simulink model "Slink__Analog_Buck_Control"  (R2023b)
settings: Solver=VariableStepAuto  StartTime=0.0  StopTime=1  RelTol=1e-6
values from neighbouring files (symbols this model uses):
  C = 22e-6    (= 2.2e-05)    [Final_Project.m]
  C2_c = 1e-6    (= 1e-06)    [Final_Project.m]
  fs = 12e3    (= 12000)    [Final_Project.m]
  L = 1e-3    (= 0.001)    [Final_Project.m]
  R = 22    [Final_Project.m]
  R1 = 20e3    (= 20000)    [Final_Project.m]
  R1_c = 10e3    (= 10000)    [Final_Project.m]
  R2 = Hs*R1    (= 2000)    [Final_Project.m]
  R3_c = 10e3    (= 10000)    [Final_Project.m]
  R4_c = 3.9e3    (= 3900)    [Final_Project.m]
  Vd = 36*sqrt(2)    [Final_Project.m]
libraries: spsSeriesRLCBranchLib x23, spsGroundLib x11, spsVoltageMeasurementLib x9, spsControlledVoltageSourceLib x6, simulink x4, spsCurrentMeasurementLib x1, spsDiodeLib x1, spsIdealSwitchLib x1, spsMeanLib x1, eePwmGenerator x1, spspowerguiLib x1
settings Model: Creator=Lucas  LastModifiedBy=Lucas

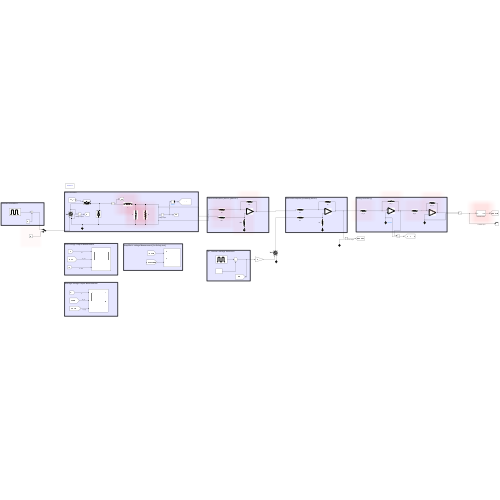
[thumbnail: Simulink's stored preview of the top-level diagram]
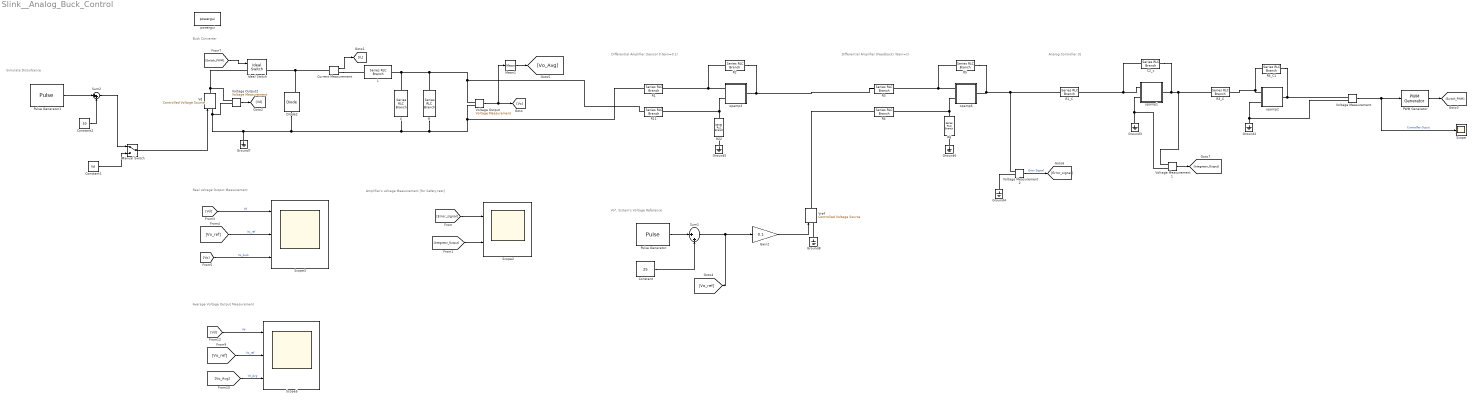
== system Slink__Analog_Buck_Control ==
  note: Amplifier's voltage Measurement [for Safety test]
  note: Vo*, Sistem's Voltage Reference
  note: Simulate Disturbance
  note: Differential Amplifier [Feedback] (Gain=1)
  note: Analog Controller [I]
  note: Differential Amplifier [Sensor ](Gain=0.1)
  note: Buck Converter
  note: Average Voltage Output Measurement
  note: Real voltage Output Measurement
  C : spsSeriesRLCBranchLib/Series RLC Branch  LConnTagsString=__new0  RConnTagsString=__new0  BranchType=C  Resistance=1  Inductance=L  SetiL0=off  InitialCurrent=0  Capacitance=C  Setx0=off  InitialVoltage=0  Measurements=None
  C2_c : spsSeriesRLCBranchLib/Series RLC Branch  LConnTagsString=__new0  RConnTagsString=__new0  BranchType=C  Resistance=R2  Inductance=1e-3  SetiL0=off  InitialCurrent=0  Capacitance=C2_c  Setx0=off  InitialVoltage=0  Measurements=None
  Constant : Constant  Value=25
  Constant1 : Constant  Value=Vd
  Constant2 : Constant  Value=50
  Current Measurement : spsCurrentMeasurementLib/Current Measurement  PhasorSimulation=off  OutputType=Complex  PSBequivalent=0
  Diode2 : spsDiodeLib/Diode  Ron=0.00001  Lon=0  Vf=0  IC=0  UseSnubber=0  Rs=inf  Cs=inf  Measurements=on
  Gain2 : Gain  Gain=0.1
  Ground{2..8} (7 alike) : spsGroundLib/Ground  LConnTagsString=a
  Ideal Switch : spsIdealSwitchLib/Ideal Switch  Ron=0.001  Lon=0  IC=0  Rs=1e5  Cs=inf  Measurements=on
  L : spsSeriesRLCBranchLib/Series RLC Branch  LConnTagsString=__new0  RConnTagsString=__new0  BranchType=L  Resistance=1  Inductance=L  SetiL0=off  InitialCurrent=0  Capacitance=1e-6  Setx0=off  InitialVoltage=0  Measurements=None
  Manual Switch : ManualSwitch
  Mean1 : spsMeanLib/Mean  Freq=60  Vinit=0  Ts=0
  PWM Generator : eePwmGenerator/PWM Generator  CarrCount=Up  Tper=1/fs  Tdelay=0  Ts=0
  Pulse Generator : DiscretePulseGenerator  PulseType=Time based  Amplitude=20  Period=0.5  PulseWidth=50  PhaseDelay=0.2
  Pulse Generator1 : DiscretePulseGenerator  PulseType=Time based  Amplitude=20  Period=0.5  PulseWidth=50  PhaseDelay=0.1
  R : spsSeriesRLCBranchLib/Series RLC Branch  LConnTagsString=__new0  RConnTagsString=__new0  BranchType=R  Resistance=R  Inductance=L  SetiL0=off  InitialCurrent=0  Capacitance=1e-6  Setx0=off  InitialVoltage=0  Measurements=None
  R1 : spsSeriesRLCBranchLib/Series RLC Branch  LConnTagsString=__new0  RConnTagsString=__new0  BranchType=R  Resistance=R1  Inductance=1e-3  SetiL0=off  InitialCurrent=0  Capacitance=1e-6  Setx0=off  InitialVoltage=0  Measurements=None
  R11 : spsSeriesRLCBranchLib/Series RLC Branch  LConnTagsString=__new0  RConnTagsString=__new0  BranchType=R  Resistance=R1  Inductance=1e-3  SetiL0=off  InitialCurrent=0  Capacitance=1e-6  Setx0=off  InitialVoltage=0  Measurements=None
  R1_C : spsSeriesRLCBranchLib/Series RLC Branch  LConnTagsString=__new0  RConnTagsString=__new0  BranchType=R  Resistance=R1_c  Inductance=1e-3  SetiL0=off  InitialCurrent=0  Capacitance=1e-6  Setx0=off  InitialVoltage=0  Measurements=None
  R2 : spsSeriesRLCBranchLib/Series RLC Branch  LConnTagsString=__new0  RConnTagsString=__new0  BranchType=R  Resistance=R2  Inductance=1e-3  SetiL0=off  InitialCurrent=0  Capacitance=1e-6  Setx0=off  InitialVoltage=0  Measurements=None
  R22 : spsSeriesRLCBranchLib/Series RLC Branch  LConnTagsString=__new0  RConnTagsString=__new0  BranchType=R  Resistance=R2  Inductance=1e-3  SetiL0=off  InitialCurrent=0  Capacitance=1e-6  Setx0=off  InitialVoltage=0  Measurements=None
  R{3..6} (4 alike) : spsSeriesRLCBranchLib/Series RLC Branch  LConnTagsString=__new0  RConnTagsString=__new0  BranchType=R  Resistance=2e3  Inductance=1e-3  SetiL0=off  InitialCurrent=0  Capacitance=1e-6  Setx0=off  InitialVoltage=0  Measurements=None
  R3_C : spsSeriesRLCBranchLib/Series RLC Branch  LConnTagsString=__new0  RConnTagsString=__new0  BranchType=R  Resistance=R3_c  Inductance=1e-3  SetiL0=off  InitialCurrent=0  Capacitance=1e-6  Setx0=off  InitialVoltage=0  Measurements=None
  R4_C1 : spsSeriesRLCBranchLib/Series RLC Branch  LConnTagsString=__new0  RConnTagsString=__new0  BranchType=R  Resistance=R4_c  Inductance=1e-3  SetiL0=off  InitialCurrent=0  Capacitance=1e-6  Setx0=off  InitialVoltage=0  Measurements=None
  Scope : Scope
  Scope2 : Scope  NumInputPorts=2
  Scope3 : Scope  NumInputPorts=3
  Scope5 : Scope  NumInputPorts=3
  Sum1 : Sum  Inputs=|++
  Sum2 : Sum  Inputs=|++
  Vd : spsControlledVoltageSourceLib/Controlled Voltage Source  Initialize=on  Source_Type=DC  Amplitude=50  Phase=0  Frequency=0  Measurements=None
  Voltage Measurement : spsVoltageMeasurementLib/Voltage Measurement  PhasorSimulation=off  OutputType=Complex  PSBequivalent=0
  Voltage Measurement1 : spsVoltageMeasurementLib/Voltage Measurement  PhasorSimulation=off  OutputType=Complex  PSBequivalent=0
  Voltage Measurement2 : spsVoltageMeasurementLib/Voltage Measurement  PhasorSimulation=off  OutputType=Complex  PSBequivalent=0
  Voltage Output : spsVoltageMeasurementLib/Voltage Measurement  PhasorSimulation=off  OutputType=Complex  PSBequivalent=0
  Voltage Output2 : spsVoltageMeasurementLib/Voltage Measurement  PhasorSimulation=off  OutputType=Complex  PSBequivalent=0
  Vref : spsControlledVoltageSourceLib/Controlled Voltage Source  Initialize=on  Source_Type=DC  Amplitude=0  Phase=0  Frequency=0  Measurements=None
  opamp1 : Subsystem  mask(Opamp){Ri=1e7, Ro=100, A=200000, U1=12, U2=-12}
      mask prompts: Ri "Input Resistance"; Ro "Output Resistance"; A "Open loop amplification"; U1 "Upper limit supply voltage"; U2 "Lower limit supply voltage"
      mask Display:
      | plot([10 20 30 40], [10 12 14 16],[10 20 30 40], [22 20 18 16],[10 10],[10 22])
      | text(10,13.4,'+')
      | text(10,21,'_')
  opamp2 : Subsystem  mask(Opamp){Ri=1e7, Ro=100, A=200000, U1=12, U2=-12}
      mask prompts: Ri "Input Resistance"; Ro "Output Resistance"; A "Open loop amplification"; U1 "Upper limit supply voltage"; U2 "Lower limit supply voltage"
      mask Display:
      | plot([10 20 30 40], [10 12 14 16],[10 20 30 40], [22 20 18 16],[10 10],[10 22])
      | text(10,13.4,'+')
      | text(10,21,'_')
  opamp3 : Subsystem  mask(Opamp){Ri=1e7, Ro=100, A=200000, U1=12, U2=-12}
      mask prompts: Ri "Input Resistance"; Ro "Output Resistance"; A "Open loop amplification"; U1 "Upper limit supply voltage"; U2 "Lower limit supply voltage"
      mask Display:
      | plot([10 20 30 40], [10 12 14 16],[10 20 30 40], [22 20 18 16],[10 10],[10 22])
      | text(10,13.4,'+')
      | text(10,21,'_')
  opamp6 : Subsystem  mask(Opamp){Ri=1e7, Ro=100, A=200000, U1=12, U2=-12}
      mask prompts: Ri "Input Resistance"; Ro "Output Resistance"; A "Open loop amplification"; U1 "Upper limit supply voltage"; U2 "Lower limit supply voltage"
      mask Display:
      | plot([10 20 30 40], [10 12 14 16],[10 20 30 40], [22 20 18 16],[10 10],[10 22])
      | text(10,13.4,'+')
      | text(10,21,'_')
  powergui : spspowerguiLib/powergui  Priority=1  SimulationMode=Continuous  SampleTime=50e-6  frequency=60  Iterations=50  frequencyindice=0  Pbase=100e6  ErrMax=1e-4  UnitsV=kV  UnitsW=MW  buscounter=0  FunctionMessages=off  echomessages=off  EnableUseOfTLC=off  CurrentSourceSwitches=off  DisableSnubberDevices=off  DisableRonSwitches=off  DisableVfSwitches=off  DisplayEquations=off  AutomaticDiscreteSolvers=off  SolverType=Tustin/Backward Euler (TBE)  Interpol=off  ExternalGateDelay=off  methode=off  Ts=100  x0status=blocks  SPID=on  SwTol=0  HookPort=off  NonlinearTolerance=1e-4  nMaxIteration=100  ContinueOnMaxIteration=off  RestoreLinks=warning  ResistiveCurrentMeasurement=off  Frange=[0:2:500]  Ylog=off  Xlog=on  ShowGrid=off  save=off  variable=ZData  structure=0  ZoomFFT=off  StartTime=0.0  cycles=1  DisplayStyle=1  fundamental=60  FreqAxis=off  MaxFrequency=1000  frequencyindicesteady=1  RmsSteady=1  display=off
  wires:
  Constant1/1 -> Manual Switch/2
  Voltage Output2/1 -> [Vd]
  Manual Switch/1 -> Vd/1
  Mean1/1 -> [Vo_Avg]
  Voltage Output/1 -> Mean1/1, [Vo]
  Pulse Generator1/1 -> Sum2/1
  Sum2/1 -> Manual Switch/1
  [Switch_PWM] -> Ideal Switch/1
  Current Measurement/1 -> [IL]
  Constant2/1 -> Sum2/2
  Pulse Generator/1 -> Sum1/1
  Constant/1 -> Sum1/2
  Sum1/1 -> Gain2/1, [Vo_ref]
  Voltage Measurement/1 -> Scope/1, PWM Generator/1  "Controlller Ouput"
  PWM Generator/1 -> [Switch_PWM]
  [Vo_ref] -> Scope5/2  "Vo_ref"
  [Vo_Avg] -> Scope5/3  "Vo_Avg"
  [Vd] -> Scope5/1  "Vd"
  Gain2/1 -> Vref/1
  [Vo] -> Scope3/3  "Vo_buck"
  [Vo_ref] -> Scope3/2  "Vo_ref"
  [Vd] -> Scope3/1  "Vd"
  Voltage Measurement2/1 -> [Error_signal]  "Error Signal"
  Voltage Measurement1/1 -> [Integrator_Output]
  [Integrator_Output] -> Scope2/2
  [Error_signal] -> Scope2/1
  connections:
  R1_C/LConn1 -- Voltage Measurement2/LConn1 -- opamp6/RConn1 -- R5/RConn1
  opamp2/LConn1 -- R3_C/RConn1 -- R4_C1/LConn1
  R4/RConn1 -- R6/LConn1 -- opamp6/LConn2
  opamp1/RConn1 -- Voltage Measurement1/LConn1 -- R3_C/LConn1 -- C2_c/RConn1
  opamp3/LConn1 -- R2/LConn1 -- R1/RConn1
  opamp6/LConn1 -- R3/RConn1 -- R5/LConn1
  R1_C/RConn1 -- C2_c/LConn1 -- opamp1/LConn1
  R11/RConn1 -- opamp3/LConn2 -- R22/LConn1
  R2/RConn1 -- R3/LConn1 -- opamp3/RConn1
  Ground6/LConn1 -- R6/RConn1
  opamp1/LConn2 -- Voltage Measurement1/LConn2 -- Ground3/LConn1
  R4_C1/RConn1 -- Voltage Measurement/LConn1 -- opamp2/RConn1
  Ground5/LConn1 -- R22/RConn1
  opamp2/LConn2 -- Voltage Measurement/LConn2 -- Ground2/LConn1
  Diode2/RConn1 -- Ideal Switch/RConn1 -- Current Measurement/LConn1
  Voltage Output2/LConn1 -- Ideal Switch/LConn1 -- Vd/RConn1
  C/LConn1 -- L/RConn1 -- Voltage Output/LConn1 -- R11/LConn1 -- R/LConn1
  Vd/LConn1 -- Ground7/LConn1 -- C/RConn1 -- R1/LConn1 -- Voltage Output/LConn2 -- R/RConn1 -- Diode2/LConn1 -- Voltage Output2/LConn2
  Current Measurement/RConn1 -- L/LConn1
  Vref/RConn1 -- R4/LConn1
  Ground8/LConn1 -- Vref/LConn1
  Ground4/LConn1 -- Voltage Measurement2/LConn2

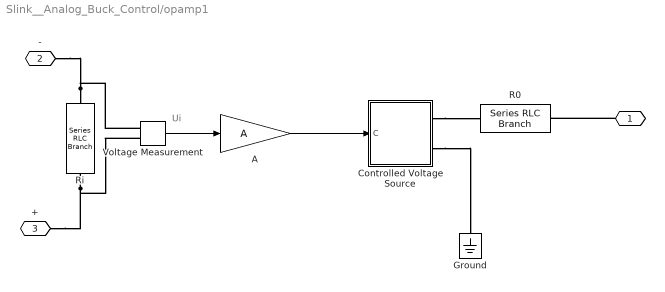
== system Slink__Analog_Buck_Control/opamp1 ==
  note: Ui
  A : Gain  Gain=A
  Controlled Voltage Source : Subsystem
  Ground : spsGroundLib/Ground  LConnTagsString=a
  R0 : spsSeriesRLCBranchLib/Series RLC Branch  LConnTagsString=__new0  RConnTagsString=__new0  BranchType=R  Resistance=Ro  Inductance=1.0  SetiL0=off  InitialCurrent=0  Capacitance=1.0  Setx0=off  InitialVoltage=0  Measurements=None
  Ri : spsSeriesRLCBranchLib/Series RLC Branch  LConnTagsString=__new0  RConnTagsString=__new0  BranchType=R  Resistance=Ri  Inductance=1.0  SetiL0=off  InitialCurrent=0  Capacitance=1.0  Setx0=off  InitialVoltage=0  Measurements=None
  Voltage Measurement : spsVoltageMeasurementLib/Voltage Measurement  PhasorSimulation=off  OutputType=Complex  PSBequivalent=0
  " " : PMIOPort  Side=Right
  - : PMIOPort  Port=2  Side=Left
  + : PMIOPort  Port=3  Side=Left
  wires:
  A/1 -> Controlled Voltage Source/1(C)
  Voltage Measurement/1 -> A/1
  connections:
  Controlled Voltage Source/RConn2 -- Ground/LConn1
  Ri/RConn1 -- Voltage Measurement/LConn2 -- +/RConn1
  Ri/LConn1 -- Voltage Measurement/LConn1 -- -/RConn1
  Controlled Voltage Source/RConn1 -- R0/RConn1
  " "/RConn1 -- R0/LConn1

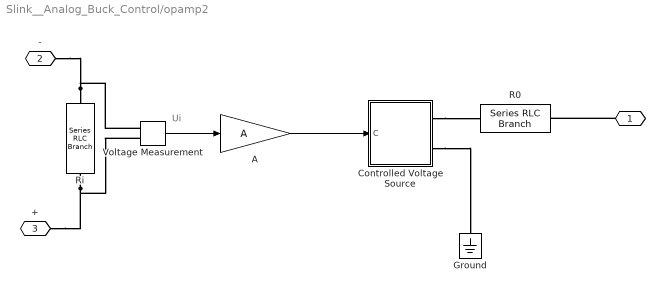
== system Slink__Analog_Buck_Control/opamp2 ==
  note: Ui
  A : Gain  Gain=A
  Controlled Voltage Source : Subsystem
  Ground : spsGroundLib/Ground  LConnTagsString=a
  R0 : spsSeriesRLCBranchLib/Series RLC Branch  LConnTagsString=__new0  RConnTagsString=__new0  BranchType=R  Resistance=Ro  Inductance=1.0  SetiL0=off  InitialCurrent=0  Capacitance=1.0  Setx0=off  InitialVoltage=0  Measurements=None
  Ri : spsSeriesRLCBranchLib/Series RLC Branch  LConnTagsString=__new0  RConnTagsString=__new0  BranchType=R  Resistance=Ri  Inductance=1.0  SetiL0=off  InitialCurrent=0  Capacitance=1.0  Setx0=off  InitialVoltage=0  Measurements=None
  Voltage Measurement : spsVoltageMeasurementLib/Voltage Measurement  PhasorSimulation=off  OutputType=Complex  PSBequivalent=0
  " " : PMIOPort  Side=Right
  - : PMIOPort  Port=2  Side=Left
  + : PMIOPort  Port=3  Side=Left
  wires:
  A/1 -> Controlled Voltage Source/1(C)
  Voltage Measurement/1 -> A/1
  connections:
  Controlled Voltage Source/RConn2 -- Ground/LConn1
  Ri/RConn1 -- Voltage Measurement/LConn2 -- +/RConn1
  Ri/LConn1 -- Voltage Measurement/LConn1 -- -/RConn1
  Controlled Voltage Source/RConn1 -- R0/RConn1
  " "/RConn1 -- R0/LConn1

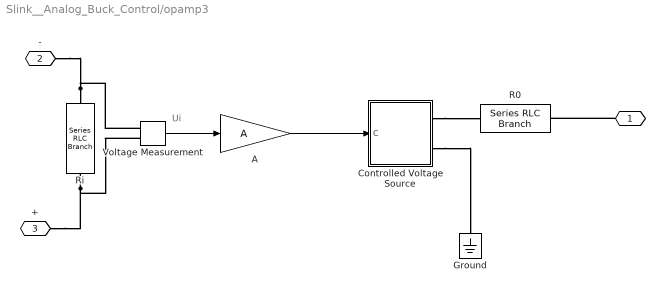
== system Slink__Analog_Buck_Control/opamp3 ==
  note: Ui
  A : Gain  Gain=A
  Controlled Voltage Source : Subsystem
  Ground : spsGroundLib/Ground  LConnTagsString=a
  R0 : spsSeriesRLCBranchLib/Series RLC Branch  LConnTagsString=__new0  RConnTagsString=__new0  BranchType=R  Resistance=Ro  Inductance=1.0  SetiL0=off  InitialCurrent=0  Capacitance=1.0  Setx0=off  InitialVoltage=0  Measurements=None
  Ri : spsSeriesRLCBranchLib/Series RLC Branch  LConnTagsString=__new0  RConnTagsString=__new0  BranchType=R  Resistance=Ri  Inductance=1.0  SetiL0=off  InitialCurrent=0  Capacitance=1.0  Setx0=off  InitialVoltage=0  Measurements=None
  Voltage Measurement : spsVoltageMeasurementLib/Voltage Measurement  PhasorSimulation=off  OutputType=Complex  PSBequivalent=0
  " " : PMIOPort  Side=Right
  - : PMIOPort  Port=2  Side=Left
  + : PMIOPort  Port=3  Side=Left
  wires:
  A/1 -> Controlled Voltage Source/1(C)
  Voltage Measurement/1 -> A/1
  connections:
  Controlled Voltage Source/RConn2 -- Ground/LConn1
  Ri/RConn1 -- Voltage Measurement/LConn2 -- +/RConn1
  Ri/LConn1 -- Voltage Measurement/LConn1 -- -/RConn1
  Controlled Voltage Source/RConn1 -- R0/RConn1
  " "/RConn1 -- R0/LConn1

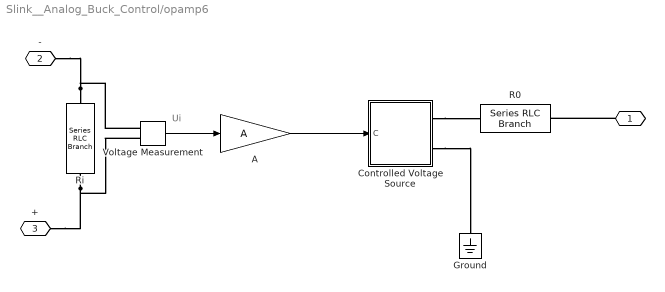
== system Slink__Analog_Buck_Control/opamp6 ==
  note: Ui
  A : Gain  Gain=A
  Controlled Voltage Source : Subsystem
  Ground : spsGroundLib/Ground  LConnTagsString=a
  R0 : spsSeriesRLCBranchLib/Series RLC Branch  LConnTagsString=__new0  RConnTagsString=__new0  BranchType=R  Resistance=Ro  Inductance=1.0  SetiL0=off  InitialCurrent=0  Capacitance=1.0  Setx0=off  InitialVoltage=0  Measurements=None
  Ri : spsSeriesRLCBranchLib/Series RLC Branch  LConnTagsString=__new0  RConnTagsString=__new0  BranchType=R  Resistance=Ri  Inductance=1.0  SetiL0=off  InitialCurrent=0  Capacitance=1.0  Setx0=off  InitialVoltage=0  Measurements=None
  Voltage Measurement : spsVoltageMeasurementLib/Voltage Measurement  PhasorSimulation=off  OutputType=Complex  PSBequivalent=0
  " " : PMIOPort  Side=Right
  - : PMIOPort  Port=2  Side=Left
  + : PMIOPort  Port=3  Side=Left
  wires:
  A/1 -> Controlled Voltage Source/1(C)
  Voltage Measurement/1 -> A/1
  connections:
  Controlled Voltage Source/RConn2 -- Ground/LConn1
  Ri/RConn1 -- Voltage Measurement/LConn2 -- +/RConn1
  Ri/LConn1 -- Voltage Measurement/LConn1 -- -/RConn1
  Controlled Voltage Source/RConn1 -- R0/RConn1
  " "/RConn1 -- R0/LConn1

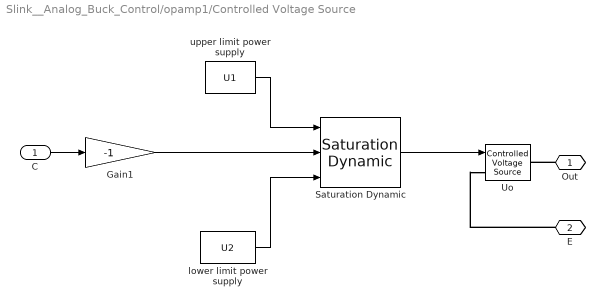
== system Slink__Analog_Buck_Control/opamp1/Controlled Voltage Source ==
  C : Inport
  Gain1 : Gain  Gain=-1
  Saturation Dynamic : simulink/Discontinuities/Saturation Dynamic  OutMin=[]  OutMax=[]  OutDataTypeStr=Inherit: Same as second input  OutDataType=fixdt(1, 16)  OutScaling=2^-10  DoSatur=off
  Uo : spsControlledVoltageSourceLib/Controlled Voltage Source  Initialize=off  Source_Type=AC  Amplitude=0  Phase=0  Frequency=0  Measurements=None
  lower limit power supply : Constant  Value=U2
  upper limit power supply : Constant  Value=U1
  Out : PMIOPort  Side=Right
  E : PMIOPort  Port=2  Side=Right
  wires:
  Gain1/1 -> Saturation Dynamic/2
  lower limit power supply/1 -> Saturation Dynamic/3
  upper limit power supply/1 -> Saturation Dynamic/1
  C/1 -> Gain1/1
  Saturation Dynamic/1 -> Uo/1
  connections:
  Out/RConn1 -- Uo/RConn1
  E/RConn1 -- Uo/LConn1

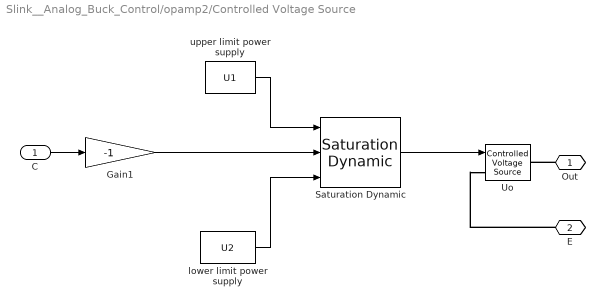
== system Slink__Analog_Buck_Control/opamp2/Controlled Voltage Source ==
  C : Inport
  Gain1 : Gain  Gain=-1
  Saturation Dynamic : simulink/Discontinuities/Saturation Dynamic  OutMin=[]  OutMax=[]  OutDataTypeStr=Inherit: Same as second input  OutDataType=fixdt(1, 16)  OutScaling=2^-10  DoSatur=off
  Uo : spsControlledVoltageSourceLib/Controlled Voltage Source  Initialize=off  Source_Type=AC  Amplitude=0  Phase=0  Frequency=0  Measurements=None
  lower limit power supply : Constant  Value=U2
  upper limit power supply : Constant  Value=U1
  Out : PMIOPort  Side=Right
  E : PMIOPort  Port=2  Side=Right
  wires:
  Gain1/1 -> Saturation Dynamic/2
  lower limit power supply/1 -> Saturation Dynamic/3
  upper limit power supply/1 -> Saturation Dynamic/1
  C/1 -> Gain1/1
  Saturation Dynamic/1 -> Uo/1
  connections:
  Out/RConn1 -- Uo/RConn1
  E/RConn1 -- Uo/LConn1

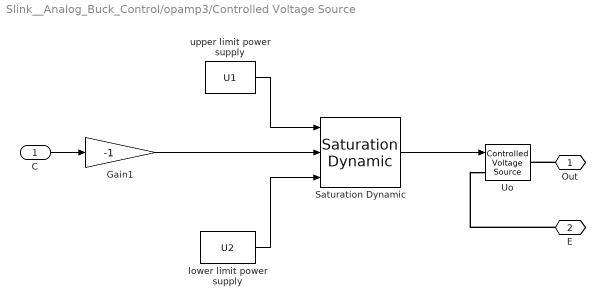
== system Slink__Analog_Buck_Control/opamp3/Controlled Voltage Source ==
  C : Inport
  Gain1 : Gain  Gain=-1
  Saturation Dynamic : simulink/Discontinuities/Saturation Dynamic  OutMin=[]  OutMax=[]  OutDataTypeStr=Inherit: Same as second input  OutDataType=fixdt(1, 16)  OutScaling=2^-10  DoSatur=off
  Uo : spsControlledVoltageSourceLib/Controlled Voltage Source  Initialize=off  Source_Type=AC  Amplitude=0  Phase=0  Frequency=0  Measurements=None
  lower limit power supply : Constant  Value=U2
  upper limit power supply : Constant  Value=U1
  Out : PMIOPort  Side=Right
  E : PMIOPort  Port=2  Side=Right
  wires:
  Gain1/1 -> Saturation Dynamic/2
  lower limit power supply/1 -> Saturation Dynamic/3
  upper limit power supply/1 -> Saturation Dynamic/1
  C/1 -> Gain1/1
  Saturation Dynamic/1 -> Uo/1
  connections:
  Out/RConn1 -- Uo/RConn1
  E/RConn1 -- Uo/LConn1

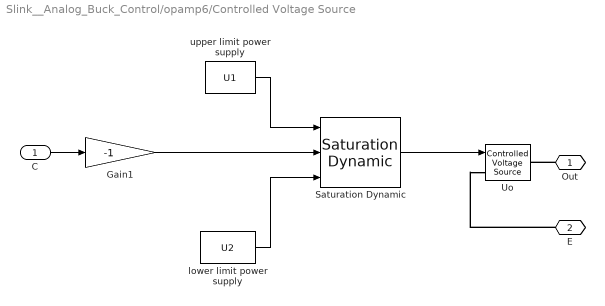
== system Slink__Analog_Buck_Control/opamp6/Controlled Voltage Source ==
  C : Inport
  Gain1 : Gain  Gain=-1
  Saturation Dynamic : simulink/Discontinuities/Saturation Dynamic  OutMin=[]  OutMax=[]  OutDataTypeStr=Inherit: Same as second input  OutDataType=fixdt(1, 16)  OutScaling=2^-10  DoSatur=off
  Uo : spsControlledVoltageSourceLib/Controlled Voltage Source  Initialize=off  Source_Type=AC  Amplitude=0  Phase=0  Frequency=0  Measurements=None
  lower limit power supply : Constant  Value=U2
  upper limit power supply : Constant  Value=U1
  Out : PMIOPort  Side=Right
  E : PMIOPort  Port=2  Side=Right
  wires:
  Gain1/1 -> Saturation Dynamic/2
  lower limit power supply/1 -> Saturation Dynamic/3
  upper limit power supply/1 -> Saturation Dynamic/1
  C/1 -> Gain1/1
  Saturation Dynamic/1 -> Uo/1
  connections:
  Out/RConn1 -- Uo/RConn1
  E/RConn1 -- Uo/LConn1
